simulink model "trajarduino"  (R2016b)
settings: Solver=VariableStepAuto  StartTime=0.0  StopTime=13  RelTol=1e-3
libraries: roblocks x1
settings Model: Creator=juan  LastModifiedBy=juan

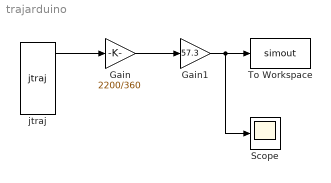
== system trajarduino ==
  Gain : Gain  Gain=2200/360
  Gain1 : Gain  Gain=57.3
  Scope : Scope
  To Workspace : ToWorkspace  VariableName=simout  SampleTime=-1
  jtraj : roblocks/Toolbox/jtraj  q0=[0 0 0]  qf=[pi/2 -pi/2 pi/2]  tmax=12  ts=0.05
  wires:
  jtraj/1 -> Gain/1
  Gain/1 -> Gain1/1
  Gain1/1 -> Scope/1, To Workspace/1
